simulink model "simulering_vinkel"  (R2017a)
settings: Solver=VariableStepAuto  StartTime=0.0  StopTime=40000  RelTol=1e-3  EnableMultiTasking=on
values from neighbouring files (symbols this model uses):
  Ad = 0.606534330298    [sysd.mat]    (also in trock.m = sysd.A)
  Bd = [-0.0242754206752 -0.00855612972972]    [sysd.mat]    (also in trock.m = [ sysd.B(5) sysd.B(6) ])
  Cd = [0.128107607141 0.111213837289]    [sysd.mat]    (also in trock.m = [ sysd.C(2); sysd.C(4) ])
  Dd = [-0.0321285947629  0.0590346867599; -0.035674975325  0.0556784277831]    [sysd.mat]    (also in trock.m = [ sysd.D(2,5) sysd.D(2,6); sysd.D(4,5) sysd.D(4,6) ])
  Ed = [ sysd.B(2) sysd.B(4)]    [trock.m]
  Kd = [ sysd.D(2,2) sysd.D(2,4); sysd.D(4,2) sysd.D(4,4) ]    [trock.m]
  Ts = 6.4385    [sysd.mat]    (also in trock.m = 600)
libraries: powerlib_meascontrol x1
settings Model: Creator=Trojass  LastModifiedBy=nvink
settings OptimizationCC: LifeSpan=inf
settings DebuggingCC: SFUnexpectedBacktrackingDiag=warning  SFNoUnconditionalDefaultTransitionDiag=warning  SFExecutionAtInitializationDiag=none
settings GRTTargetCC: TargetLangStandard=C89/C90 (ANSI)  GeneratePreprocessorConditionals=Disable all
settings ConfigComp: CovMetricSettings=dw  CovHtmlReporting=on  CovSaveCumulativeToWorkspaceVar=on  CovSaveSingleToWorkspaceVar=on  CovExternalEMLEnable=off

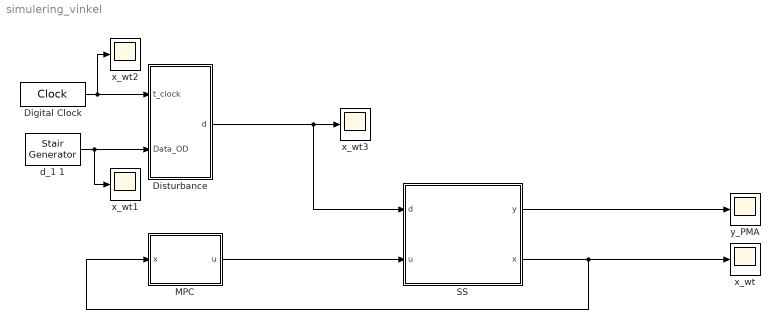
== system simulering_vinkel ==
  Digital Clock : DigitalClock  SampleTime=Ts
  "Disturbance " : MATLAB Function  TreatAsAtomicUnit=on
  MPC : MATLAB Function  TreatAsAtomicUnit=on
  SS : Subsystem
  d_1 1 : powerlib_meascontrol/Pulse & Signal Generators/Stair Generator  t=t_1  e=Data_OD  Ts=Ts
      settings: SourceProductName=Simscape Power Systems
  x_wt{,1..3} (4 alike) : Scope
  y_PMA : Scope
  wires:
  SS/1(y) -> y_PMA/1
  SS/2(x) -> MPC/1(x), x_wt/1
  Digital Clock/1 -> x_wt2/1, "Disturbance "/1(t_clock)
  "Disturbance "/1(d) -> x_wt3/1, SS/1(d)
  d_1 1/1 -> x_wt1/1, "Disturbance "/2(Data_OD)
  MPC/1(u) -> SS/2(u)

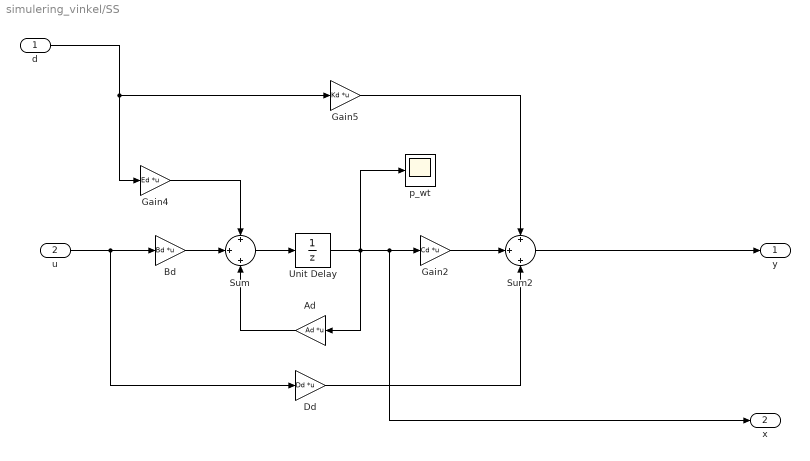
== system simulering_vinkel/SS ==
  d : Inport
  u : Inport  Port=2
  Ad : Gain  Gain=Ad  Multiplication=Matrix(K*u)
      mask Display:
      | %color('cyan')
      | color('magenta')
      | disp('{\bf\fontsize{14}Ad}', 'texmode','on');
      | %disp('Ad')
  Bd : Gain  Gain=Bd  Multiplication=Matrix(K*u)
      mask Display:
      | %color('cyan')
      | color('magenta')
      | disp('{\bf\fontsize{14}Bd}', 'texmode','on');
      | %disp('Bd')
  Dd : Gain  Gain=Dd  Multiplication=Matrix(K*u)
      mask Display:
      | %color('cyan')
      | color('magenta')
      | disp('{\bf\fontsize{14}Dd}', 'texmode','on');
      | %disp('Dd')
  Gain2 : Gain  Gain=Cd  Multiplication=Matrix(K*u)
      mask Display:
      | %color('cyan')
      | color('magenta')
      | disp('{\bf\fontsize{14}Cd}', 'texmode','on');
      | %disp('Cd')
  Gain4 : Gain  Gain=Ed  Multiplication=Matrix(K*u)
      mask Display:
      | %color('cyan')
      | color('magenta')
      | disp('{\bf\fontsize{14}Ed}', 'texmode','on');
      | %disp('Ed')
  Gain5 : Gain  Gain=Kd  Multiplication=Matrix(K*u)
      mask Display:
      | %color('cyan')
      | color('magenta')
      | disp('{\bf\fontsize{14}Kd}', 'texmode','on');
      | %disp('Kd')
  Sum : Sum  Inputs=+|+|+
  Sum2 : Sum  Inputs=+|+|+
  Unit Delay : UnitDelay  SampleTime=Ts
  p_wt : Scope
  y : Outport
  x : Outport  Port=2
  wires:
  Sum2/1 -> y/1
  Sum/1 -> Unit Delay/1
  Bd/1 -> Sum/2
  Ad/1 -> Sum/3
  Unit Delay/1 -> p_wt/1, x/1, Gain2/1, Ad/1
  u/1 -> Dd/1, Bd/1
  d/1 -> Gain4/1, Gain5/1
  Gain4/1 -> Sum/1
  Gain2/1 -> Sum2/2
  Dd/1 -> Sum2/3
  Gain5/1 -> Sum2/1

== matlab function simulering_vinkel/Disturbance  ==
  data: t_clock input; d output; Data_OD input
function d   = fcn(t_clock, Data_OD)

d_intt = load('Disturbance_Plot.mat');

d_int =[d_intt.Data_OD d_intt.Data_OD]

t_h = 1+floor(t_clock/3600);
if t_h ~= 24  
    t_int  = t_h - floor(t_h/24)*24;
else
    t_int = 24;
end

d = d_int(t_int,:)';

== matlab function simulering_vinkel/MPC ==
  data: x input; u output
function u  = fcn(x)

u = [x*10 x*2]';
end
